simulink model "TVCRocketSimulation"  (R2021a)
settings: Solver=VariableStepAuto  StartTime=0.0  StopTime=10  RelTol=1e-3
libraries: simulink_extras x3, pid_lib x1, shared3dof x1, simulink x1
settings Model: Creator=ian  LastModifiedBy=elija

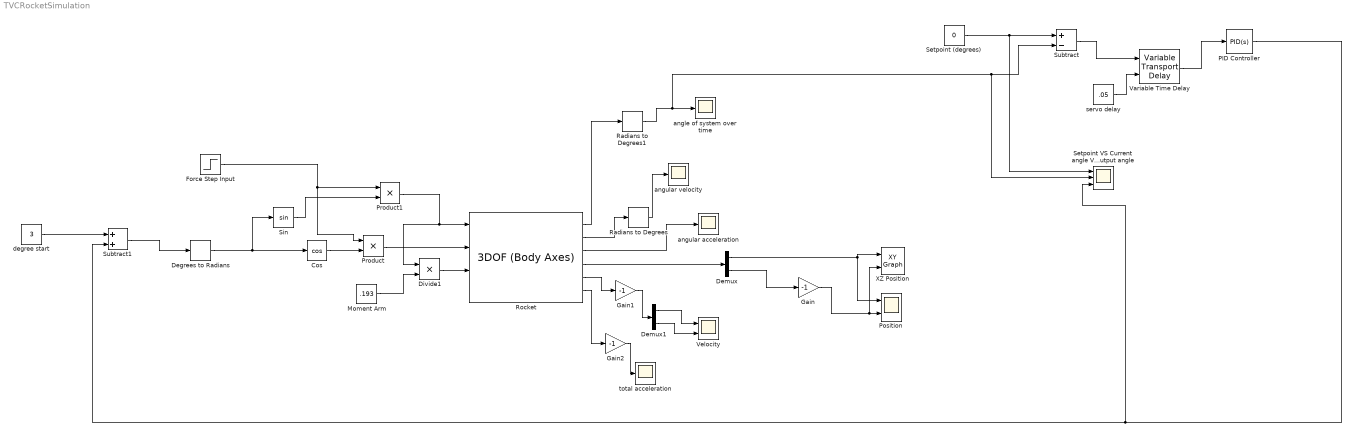
== system TVCRocketSimulation ==
  Cos : Trigonometry  Operator=cos
  Degrees to Radians : simulink_extras/Transformations/Degrees to Radians
  Demux : Demux  Outputs=2
  Demux1 : Demux  Outputs=2
  Divide1 : Product  Inputs=**
  Force Step Input : Step  Time=2.4  Before=-15  After=0
  Gain : Gain  Gain=-1
  Gain1 : Gain  Gain=-1
  Gain2 : Gain  Gain=-1
  Moment Arm : Constant  Value=.193
  PID Controller : pid_lib/PID Controller  Controller=PID  Form=Parallel  TimeDomain=Continuous-time  UseExternalTs=off  SampleTime=-1  IntegratorMethod=Forward Euler  FilterMethod=Forward Euler  ControllerParametersSource=internal  P=.35  I=0  D=.08  UseFilter=on  N=100  TunerSelectOption=Transfer Function Based (PID Tuner App)  InitialConditionSource=internal  InitialConditionForIntegrator=0  InitialConditionForFilter=0  DifferentiatorICPrevScaledInput=0  ExternalReset=none  TrackingMode=off  Kt=1  LimitOutput=on  SatLimitsSource=internal  UpperSaturationLimit=5  LowerSaturationLimit=-5  LinearizeAsGain=on  AntiWindupMode=none  Kb=1  POutMin=[]  POutMax=[]  IOutMin=[]  IOutMax=[]  DOutMin=[]  DOutMax=[]  NOutMin=[]  NOutMax=[]  SumOutMin=[]  SumOutMax=[]  SaturationOutMin=[]  SaturationOutMax=[]  PParamMin=[]  PParamMax=[]  IParamMin=[]  IParamMax=[]  DParamMin=[]  DParamMax=[]  NParamMin=[]  NParamMax=[]  KbParamMin=[]  KbParamMax=[]  KtParamMin=[]  KtParamMax=[]  KbOutMin=[]  KbOutMax=[]  KtOutMin=[]  KtOutMax=[]  IntegratorOutMin=[]  IntegratorOutMax=[]  FilterOutMin=[]  FilterOutMax=[]  SumI1OutMin=[]  SumI1OutMax=[]  SumI2OutMin=[]  SumI2OutMax=[]  SumI3OutMin=[]  SumI3OutMax=[]  SumI4OutMin=[]  SumI4OutMax=[]  SumDOutMin=[]  SumDOutMax=[]  DifferentiatorOutMin=[]  DifferentiatorOutMax=[]  FilterDiffOutCoefMin=[]  FilterDiffOutCoefMax=[]  ReciprocalOutMin=[]  ReciprocalOutMax=[]  SumDenOutMin=[]  SumDenOutMax=[]  SumNumOutMin=[]  SumNumOutMax=[]  DivideOutMin=[]  DivideOutMax=[]  UdiffTsProdOutMin=[]  UdiffTsProdOutMax=[]  NTsProdOutMin=[]  NTsProdOutMax=[]  UintegralTsProdOutMin=[]  UintegralTsProdOutMax=[]  UngainTsProdOutMin=[]  UngainTsProdOutMax=[]  IntegratorContinuousStateAttributes=''  IntegratorStateMustResolveToSignalObject=off  IntegratorRTWStateStorageClass=Auto  FilterContinuousStateAttributes=''  FilterStateMustResolveToSignalObject=off  FilterRTWStateStorageClass=Auto  ParallelPVariant=InternalParameters  IdealPVariant=Disabled  IVariant=InternalParameters  DVariant=InternalParameters  IntegratorVariant=Continuous  SatVariant=Enabled  AWVariant=Passthrough  PCopyVariant=Disabled  TRVariant=Disabled  FdbkBlocksVariant=Forward  IdealPFdbkVariant=Disabled  SatFdbkVariant=Disabled  DerivativeFilterVariant=ContFilter  NVariant=InternalParameters  NCopyVariant=Disabled  FilterICVariant=InternalICsFilter  IntegratorICVariant=InternalICs  ExternalResetVariant=Disabled  TRSumVariant=Passthrough  SumFdbkVariant=Disabled  SumVariant=Sum_PID  TsampFilterVariant=InternalTs  TsampNgainVariant=Passthrough  TsampIntegralVariant=Passthrough  ExternalSaturationOutDataTypeStr=Inherit: Same as second input
  Position : Scope  NumInputPorts=2
  Product : Product  RndMeth=Zero
  Product1 : Product  RndMeth=Zero
  Radians to Degrees : simulink_extras/Transformations/Radians to Degrees
  Radians to Degrees1 : simulink_extras/Transformations/Radians to Degrees
  Rocket : shared3dof/3DOF (Body Axes)  units=Metric (MKS)  mtype=Fixed  v_ini=0  theta_ini=0  alpha_ini=0  pos_ini=[0 0]  q_ini=0  mass=.805  mass_e=0.5  mass_f=3.0  Iyy=.017  Iyy_e=0.5  Iyy_f=3.0  g_in=External  g=9.81  vre_flag=on  abi_flag=off  aMode=0  vel_statename=''  theta_statename=''  pos_statename=''  q_statename=''  mass_statename=''
      settings: SourceProductBaseCode=AE,PW,DR,MT,UV,VE
  Setpoint (degrees) : Constant  Value=0
  Setpoint VS Current angle VS Output angle : Scope  NumInputPorts=3
  Sin : Trigonometry
  Subtract : Sum  Inputs=+-
  Subtract1 : Sum
  Variable Time Delay : VariableTransportDelay  MaximumDelay=10
  Velocity : Scope  NumInputPorts=2
  XZ Position : simulink/Sinks/XY Graph  xmin=-20  xmax=20  ymin=0  ymax=20  st=-1
  angle of system over time : Scope
  angular acceleration : Scope
  angular velocity : Scope
  degree start : Constant  Value=3
  servo delay : Constant  Value=.05
  total acceleration : Scope
  wires:
  Rocket/4 -> Demux/1
  Demux/1 -> XZ Position/1, Position/1
  Force Step Input/1 -> Product1/1, Product/1
  Cos/1 -> Product/2
  Product1/1 -> Rocket/1, Divide1/1
  Sin/1 -> Product1/2
  Product/1 -> Rocket/2
  Moment Arm/1 -> Divide1/2
  Degrees to Radians/1 -> Cos/1, Sin/1
  Demux/2 -> Gain/1
  Gain/1 -> XZ Position/2, Position/2
  Divide1/1 -> Rocket/3
  Rocket/1 -> Radians to Degrees1/1
  Rocket/6 -> Gain2/1
  Rocket/5 -> Gain1/1
  Demux1/1 -> Velocity/1
  Demux1/2 -> Velocity/2
  Gain1/1 -> Demux1/1
  Gain2/1 -> total acceleration/1
  Rocket/3 -> angular acceleration/1
  Rocket/2 -> Radians to Degrees/1
  Radians to Degrees1/1 -> Setpoint VS Current angle VS Output angle/2, Subtract/2, angle of system over time/1
  Radians to Degrees/1 -> angular velocity/1
  Setpoint (degrees)/1 -> Setpoint VS Current angle VS Output angle/1, Subtract/1
  Subtract/1 -> Variable Time Delay/1
  Variable Time Delay/1 -> PID Controller/1
  servo delay/1 -> Variable Time Delay/2
  PID Controller/1 -> Subtract1/2, Setpoint VS Current angle VS Output angle/3
  degree start/1 -> Subtract1/1
  Subtract1/1 -> Degrees to Radians/1
